simulink model "simulated_encoder"  (R2022b)
settings: Solver=FixedStepAuto  StartTime=0.0  StopTime=100  FixedStep=0.0001  RelTol=1e-3
libraries: fl_lib x5, simulink x4, nesl_utility x4, ee_lib x1, sdl_lib x1
settings Model: Creator=micha  LastModifiedBy=micha

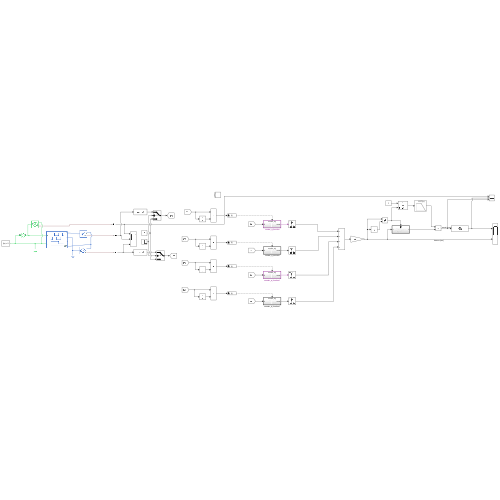
[thumbnail: Simulink's stored preview of the top-level diagram]
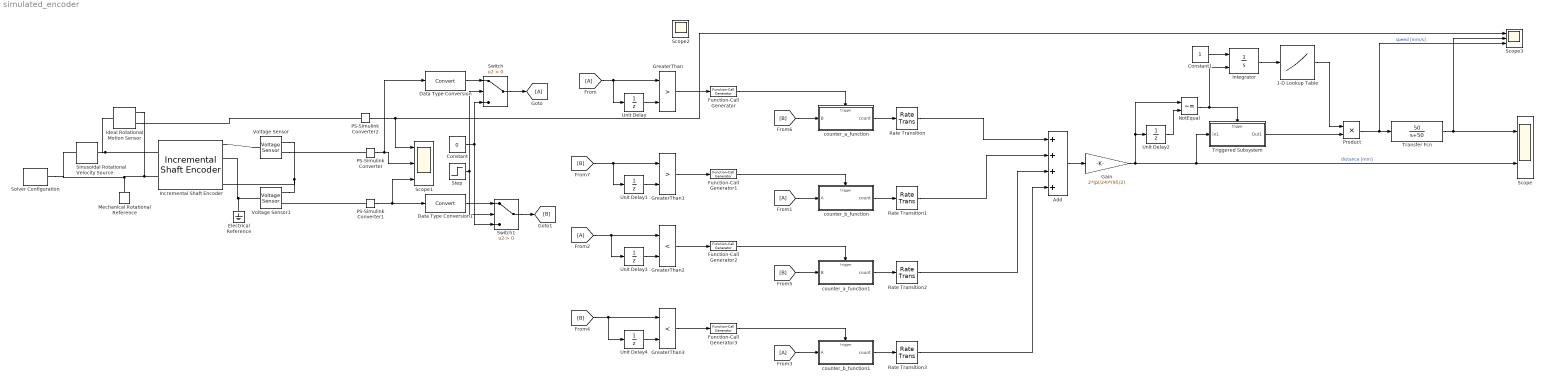
== system simulated_encoder ==
  1-D Lookup Table : Lookup_n-D  NumberOfTableDimensions=1  BreakpointsForDimension1=[0, 0.5, 1]  Table=[1, 1, 0]  ExtrapMethod=Clip  UseLastTableValue=on  InternalRulePriority=Speed  RndMeth=Simplest
  Add : Sum  Inputs=++++
  Constant : Constant  Value=0
  Constant1 : Constant
  Data Type Conversion : DataTypeConversion  SaturateOnIntegerOverflow=off  RndMeth=Floor
  Data Type Conversion1 : DataTypeConversion  SaturateOnIntegerOverflow=off  RndMeth=Floor
  Electrical Reference : fl_lib/Electrical/Electrical Elements/Electrical Reference
  From{,1..3} (4 alike) : From
  Function-Call Generator{,1..3} (4 alike) : simulink/Ports & Subsystems/Function-Call Generator  sample_time=1  numberOfIterations=1  DisallowWideOutput=off  ShowEnablePort=on
  Gain : Gain  Gain=2*(pi/24)*(95/2)
  Goto : Goto
  GreaterThan : RelationalOperator  Operator=>  OutDataTypeStr=boolean  RndMeth=Simplest  InputSameDT=off
  GreaterThan1 : RelationalOperator  Operator=>  OutDataTypeStr=boolean  RndMeth=Simplest  InputSameDT=off
  GreaterThan2 : RelationalOperator  Operator=<  OutDataTypeStr=boolean  RndMeth=Simplest  InputSameDT=off
  GreaterThan3 : RelationalOperator  Operator=<  OutDataTypeStr=boolean  RndMeth=Simplest  InputSameDT=off
  Ideal Rotational Motion Sensor : fl_lib/Mechanical/Mechanical Sensors/Ideal Rotational Motion Sensor  reference=foundation.enum.MeasurementReference.difference  acceleration_port=false  velocity_port=true  position_port=false  wrap_angle=false  offset=0 rad
      settings: InternalSimscapePortConfiguration="{\"Bottom\":[],\"Left\":[{\"id\":\"R\",\"label\":\"R\",\"type\":\"foundation.mechanical.rotational.rotational\"}],\"Right\":[{\"id\":\"C\",\"label\":\"C\",\"type\":\"foundation.mechanical.rotational.rotational\"},{\"id\":\"W\",\"label\":\"W\",\"type\":\"output\"}],\"Top\":[]}"
  Incremental Shaft Encoder : ee_lib/Sensors & Transducers/Incremental Shaft Encoder  NPulse=24  Vm=1 V  angle0=0 deg
      settings: InternalSimscapePortConfiguration="{\"Bottom\":[],\"Left\":[{\"id\":\"R\",\"label\":\"R\",\"type\":\"foundation.mechanical.rotational.rotational\"},{\"id\":\"C\",\"label\":\"C\",\"type\":\"foundation.mechanical.rotational.rotational\"}],\"Right\":[{\"id\":\"A\",\"label\":\"A\",\"type\":\"foundation.electrical.electrical\"},{\"id\":\"B\",\"label\":\"B\",\"type\":\"foundation.electrical.electrical\"},{\"id\":\"Z\",\"label\":\"Z\",\"type\":\"foundation.electrical.electrical\"},{\"id\":\"GND\",\"label\":\"REF\",\"type\":\"foundation.electrical.electrical\"}],\"Top\":[]}"
  Integrator : Integrator  ExternalReset=rising
  Mechanical Rotational Reference : fl_lib/Mechanical/Rotational Elements/Mechanical Rotational Reference
  NotEqual : RelationalOperator  Operator=~=  OutDataTypeStr=boolean  RndMeth=Simplest  InputSameDT=off
  PS-Simulink Converter : nesl_utility/PS-Simulink Converter  PhysicalDomain=network_engine_domain  SubClassName=ps_output  LeftPortType=input  RightPortType=output  PseudoPeriodic=off  Frequencies=[]  VectorFormat=inherit  Unit=inherit  AffineConversion=off
  PS-Simulink Converter1 : nesl_utility/PS-Simulink Converter  PhysicalDomain=network_engine_domain  SubClassName=ps_output  LeftPortType=input  RightPortType=output  PseudoPeriodic=off  Frequencies=[]  VectorFormat=inherit  Unit=inherit  AffineConversion=off
  PS-Simulink Converter2 : nesl_utility/PS-Simulink Converter  PhysicalDomain=network_engine_domain  SubClassName=ps_output  LeftPortType=input  RightPortType=output  PseudoPeriodic=off  Frequencies=[]  VectorFormat=inherit  Unit=inherit  AffineConversion=off
  Product : Product
  Rate Transition{,1..3} (4 alike) : RateTransition  Deterministic=off
  Scope : Scope  NumInputPorts=2
  Scope1 : Scope  NumInputPorts=3
  Scope2 : Scope  NumInputPorts=2
  Scope3 : Scope  NumInputPorts=3
  Sinusoidal Rotational Velocity Source : sdl_lib/Sources/Sinusoidal Rotational Velocity Source  offset=0 rad/s  amplitude=2*pi rad/s  phase_shift=0 deg  frequency=0.1 Hz
      settings: InternalSimscapePortConfiguration="{\"Bottom\":[],\"Left\":[{\"id\":\"B\",\"label\":\"B\",\"type\":\"foundation.mechanical.rotational.rotational\"}],\"Right\":[{\"id\":\"F\",\"label\":\"F\",\"type\":\"foundation.mechanical.rotational.rotational\"}],\"Top\":[]}"
  Solver Configuration : nesl_utility/Solver Configuration  PhysicalDomain=network_engine_domain  SubClassName=solver  LeftPortType=input  RightPortType=generic  Tones=[]  Harmonics=[]  SimulateNoise=off  Profile=off  UseLocalSampling=off  EnableSwitchedLinearOptims=on  FrequencyDomain=off  UseCCode=off  RelTol=0.001  AbsTol=0.001  MinStep=1e-09  ToWorkspace=off  RevertToSquareIcSolve=off  NumHomotopyIterations=100  PhasorMode=off  PhasorModeNumHarmonics=1  ConsistencySolver=NEWTON_XTOL_AFTER_FTOL  IndexReductionMethod=DerivativeReplacement  DoDC=off  ResidualTolerance=1e-09  ConsistencyTolSource=GLOBAL  ConsistencyAbsTol=0.001  ConsistencyRelTol=0.001  ConsistencyTolFactor=0.001  UseLocalSolver=off  LocalSolverChoice=NE_BACKWARD_EULER_ADVANCER  ResolveIndetEquations=on  FunctionEvalNumThread=1  LocalSolverSampleTime=0.001  DoFixedCost=off  MaxNonlinIter=3  MaxModeIter=2  ComputeImpulses=off  ImpulseIterations=2  LinearAlgebra=auto  LinearAlgebraNumThread=0  EquationFormulation=NE_TIME_EF  DelaysMemoryBudget=1024  AutomaticFiltering=on  FilteringTimeConstant=0.001  PartitionStorageMethod=AS_NEEDED  PartitionMemoryBudget=1024  PartitionMethod=ROBUST
  Step : Step  Time=12  Before=1  After=0  SampleTime=0
  Switch : Switch  Criteria=u2 > Threshold  SaturateOnIntegerOverflow=off  InputSameDT=off
  Switch1 : Switch  Criteria=u2 > Threshold  SaturateOnIntegerOverflow=off  InputSameDT=off
  Transfer Fcn : TransferFcn  Numerator=[50]  Denominator=[1 50]
  Triggered Subsystem : Subsystem  TreatAsAtomicUnit=on
  Unit Delay{,1..4} (5 alike) : UnitDelay  SampleTime=-1  HasFrameUpgradeWarning=on
  Voltage Sensor : fl_lib/Electrical/Electrical Sensors/Voltage Sensor
  Voltage Sensor1 : fl_lib/Electrical/Electrical Sensors/Voltage Sensor
  counter_a_function : Subsystem  TreatAsAtomicUnit=on
  counter_a_function1 : Subsystem  TreatAsAtomicUnit=on
  counter_b_function : Subsystem  TreatAsAtomicUnit=on
  counter_b_function1 : Subsystem  TreatAsAtomicUnit=on
  wires:
  Triggered Subsystem/1(Out1) -> Product/2
  Rate Transition1/1 -> Add/2
  Add/1 -> Gain/1
  Rate Transition/1 -> Add/1
  counter_b_function/1(count) -> Rate Transition1/1
  Gain/1 -> Triggered Subsystem/1(In1), Scope/2, NotEqual/1, Unit Delay2/1  "distance [mm]"
  counter_a_function/1(count) -> Rate Transition/1
  PS-Simulink Converter/1 -> Data Type Conversion/1, Scope1/2
  PS-Simulink Converter1/1 -> Data Type Conversion1/1, Scope1/3
  GreaterThan/1 -> Function-Call Generator/1
  Function-Call Generator/1 -> counter_a_function/Trigger
  Function-Call Generator1/1 -> counter_b_function/Trigger
  Unit Delay/1 -> GreaterThan/2
  GreaterThan1/1 -> Function-Call Generator1/1
  Unit Delay1/1 -> GreaterThan1/2
  NotEqual/1 -> Integrator/2, Triggered Subsystem/Trigger
  Unit Delay2/1 -> NotEqual/2
  Unit Delay3/1 -> GreaterThan2/2
  GreaterThan2/1 -> Function-Call Generator2/1
  [B] -> Unit Delay4/1, GreaterThan3/1
  Unit Delay4/1 -> GreaterThan3/2
  Function-Call Generator3/1 -> counter_b_function1/Trigger
  GreaterThan3/1 -> Function-Call Generator3/1
  counter_a_function1/1(count) -> Rate Transition2/1
  From2/1 -> Unit Delay3/1, GreaterThan2/1
  Function-Call Generator2/1 -> counter_a_function1/Trigger
  counter_b_function1/1(count) -> Rate Transition3/1
  Switch/1 -> Goto/1
  Data Type Conversion1/1 -> Switch1/1
  From/1 -> Unit Delay/1, GreaterThan/1
  From1/1 -> counter_b_function/1(A)
  From3/1 -> counter_b_function1/1(A)
  [B] -> counter_a_function1/1(B)
  [B] -> counter_a_function/1(B)
  [B] -> Unit Delay1/1, GreaterThan1/1
  Rate Transition2/1 -> Add/3
  Rate Transition3/1 -> Add/4
  Data Type Conversion/1 -> Switch/1
  Constant/1 -> Switch1/3, Switch/3
  Switch1/1 -> [B]
  Step/1 -> Switch/2, Switch1/2
  Constant1/1 -> Integrator/1
  Integrator/1 -> 1-D Lookup Table/1
  1-D Lookup Table/1 -> Product/1
  Product/1 -> Scope3/3, Transfer Fcn/1  "speed [mm/s]"
  PS-Simulink Converter2/1 -> Scope3/1, Scope1/1
  Transfer Fcn/1 -> Scope3/2, Scope/1
  connections:
  Sinusoidal Rotational Velocity Source/RConn1 -- Ideal Rotational Motion Sensor/LConn1 -- Incremental Shaft Encoder/LConn1
  Mechanical Rotational Reference/LConn1 -- Solver Configuration/RConn1 -- Sinusoidal Rotational Velocity Source/LConn1 -- Ideal Rotational Motion Sensor/RConn1 -- Incremental Shaft Encoder/LConn2
  Voltage Sensor/LConn1 -- Incremental Shaft Encoder/RConn1
  Voltage Sensor/RConn2 -- Voltage Sensor1/RConn2 -- Incremental Shaft Encoder/RConn4
  Voltage Sensor/RConn1 -- PS-Simulink Converter/LConn1
  Voltage Sensor1/LConn1 -- Electrical Reference/LConn1 -- Incremental Shaft Encoder/RConn2
  PS-Simulink Converter1/LConn1 -- Voltage Sensor1/RConn1
  Ideal Rotational Motion Sensor/RConn2 -- PS-Simulink Converter2/LConn1

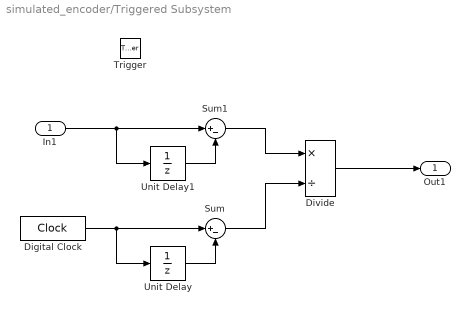
== system simulated_encoder/Triggered Subsystem ==
  In1 : Inport
  Trigger : TriggerPort  VariantControl=(inherit)
  Digital Clock : DigitalClock  SampleTime=-1
  Divide : Product  Inputs=*/
  Sum : Sum  Inputs=|+-
  Sum1 : Sum  Inputs=|+-
  Unit Delay : UnitDelay  SampleTime=-1  HasFrameUpgradeWarning=on
  Unit Delay1 : UnitDelay  SampleTime=-1  HasFrameUpgradeWarning=on
  Out1 : Outport
  wires:
  Digital Clock/1 -> Unit Delay/1, Sum/1
  Unit Delay/1 -> Sum/2
  Unit Delay1/1 -> Sum1/2
  In1/1 -> Unit Delay1/1, Sum1/1
  Sum1/1 -> Divide/1
  Sum/1 -> Divide/2
  Divide/1 -> Out1/1

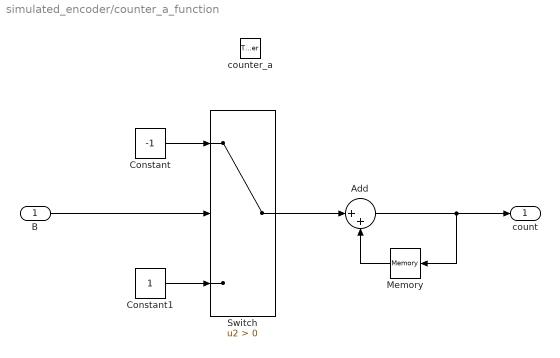
== system simulated_encoder/counter_a_function ==
  B : Inport
  counter_a : TriggerPort  TriggerType=function-call  VariantControl=(inherit)
  Add : Sum  Inputs=|++
  Constant : Constant  Value=-1
  Constant1 : Constant
  Memory : Memory  InheritSampleTime=on
  Switch : Switch  Criteria=u2 > Threshold  SaturateOnIntegerOverflow=off  InputSameDT=off
  count : Outport
  wires:
  Constant/1 -> Switch/1
  B/1 -> Switch/2
  Memory/1 -> Add/2
  Add/1 -> count/1, Memory/1
  Constant1/1 -> Switch/3
  Switch/1 -> Add/1

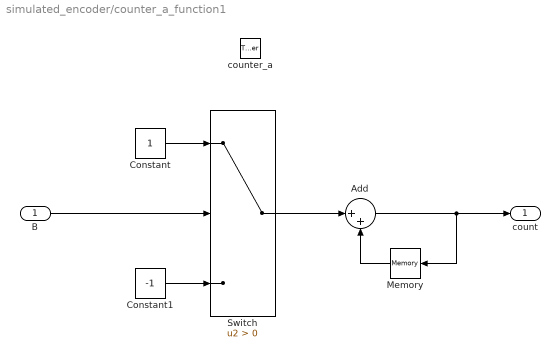
== system simulated_encoder/counter_a_function1 ==
  B : Inport
  counter_a : TriggerPort  TriggerType=function-call  VariantControl=(inherit)
  Add : Sum  Inputs=|++
  Constant : Constant
  Constant1 : Constant  Value=-1
  Memory : Memory  InheritSampleTime=on
  Switch : Switch  Criteria=u2 > Threshold  SaturateOnIntegerOverflow=off  InputSameDT=off
  count : Outport
  wires:
  Constant/1 -> Switch/1
  B/1 -> Switch/2
  Memory/1 -> Add/2
  Add/1 -> count/1, Memory/1
  Constant1/1 -> Switch/3
  Switch/1 -> Add/1

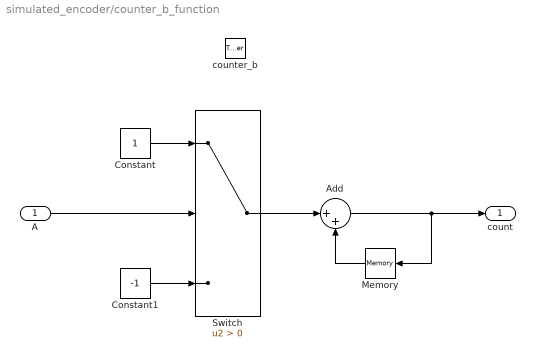
== system simulated_encoder/counter_b_function ==
  A : Inport
  counter_b : TriggerPort  TriggerType=function-call  VariantControl=(inherit)
  Add : Sum  Inputs=|++
  Constant : Constant
  Constant1 : Constant  Value=-1
  Memory : Memory  InheritSampleTime=on
  Switch : Switch  Criteria=u2 > Threshold  SaturateOnIntegerOverflow=off  InputSameDT=off
  count : Outport
  wires:
  Constant/1 -> Switch/1
  A/1 -> Switch/2
  Memory/1 -> Add/2
  Add/1 -> count/1, Memory/1
  Constant1/1 -> Switch/3
  Switch/1 -> Add/1

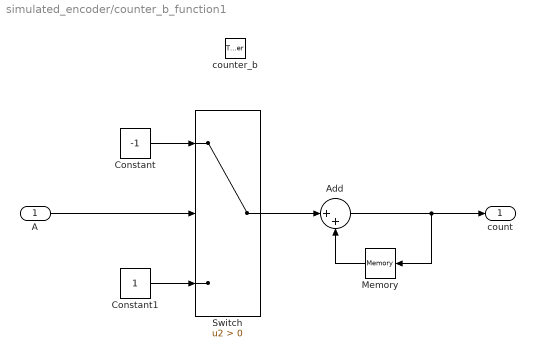
== system simulated_encoder/counter_b_function1 ==
  A : Inport
  counter_b : TriggerPort  TriggerType=function-call  VariantControl=(inherit)
  Add : Sum  Inputs=|++
  Constant : Constant  Value=-1
  Constant1 : Constant
  Memory : Memory  InheritSampleTime=on
  Switch : Switch  Criteria=u2 > Threshold  SaturateOnIntegerOverflow=off  InputSameDT=off
  count : Outport
  wires:
  Constant/1 -> Switch/1
  A/1 -> Switch/2
  Memory/1 -> Add/2
  Add/1 -> count/1, Memory/1
  Constant1/1 -> Switch/3
  Switch/1 -> Add/1
